simulink model "Car_22_Jan_test_2012b"  (R2012b)
settings: Solver=ode5  StartTime=0.0  StopTime=inf  FixedStep=sample_time  RelTol=1e-3
InitFcn:
  | sample_time=0.005;%0.004;%0.0025;%0.02;
  | sample_time_Vicon = 0.005;
  | DeltaT = 0.02;
  | g = 9.81;
  | H0 = g%0.3165;
  | Kl = 1;
  | 
  | Q6_mass = 0.84;
  | 
  | Q6_Omega_r = 1.5; %for horizon ref
  | Q6_Zeta_r = 0.5; %for horizon ref
  | Q6_Omega_r_h = 2;%for vertical ref
  | Q6_Zeta_r_h = 2; %for vertical ref
  | 
  | 
  | Q6_Omega = 1.5; %for horizon control
  | Q6_Zeta = 0.5; %for horizon control
  | Q6_Omega_h= 2; %for vertical control
  | Q6_Zeta_h = 0.7; %for vertical control
  | 
  | 
  | Q6_acc_max = 5;%horizontal max acc
  | Q6_acc_max_h = 3;%horizontal max acc
  | 
  | omega_circle = 72*pi/180;
  | omega_h = 0.1;%Ascending speed
  | PI = pi;
  | Circle_R = 2.5;
  | MAX_Height = -2;
undefined symbols (not defined in the file): DiscIntNeverNeededParam
libraries: X330_Control x5, dspswit3 x5, simulink x4
(part 2 of 2)

== matlab function Car_22_Jan_test_2012b/UAV 1/Trajectory Logic/trackbounded ==
  data: posx input; posy input; cpx input; cpy input; region output; cvx input; cvy input; newx output; newy output; newregion output; estsecond input; chkfinalx output; chkfinaly output; chknum output; directionflag output; frontbackflag output
function [region,newx,newy,newregion,chkfinalx,chkfinaly,chknum,directionflag,frontbackflag]  = fcn(posx,posy,cpx,cpy,cvx,cvy,estsecond)
%#codegen
%cp = [cpy,cpx,0];
%cpest = [estrawy, estrawx,0];
%%database of check points
chk0x = -0.4383;
chk0y = -0.9285;
chk1x = 1.047;
chk1y = -0.9693;
chk2x = 1.396;
chk2y = 0.4535;
chk3x = 1.382;
chk3y = 1.505;
chk4x = 1.042;
chk4y = 1.925;
chk5x = 0.3708;
chk5y = 1.821;
%%chk5x = ;
%%chk....
chk0 = [chk0y,chk0x,0];
chk1 = [chk1y,chk1x,0];
chk2 = [chk2y,chk2x,0];
chk3 = [chk3y,chk3x,0];
chk4 = [chk4y,chk4x,0];
chk5 = [chk5y,chk5x,0];
distance01 = sqrt((chk0y-chk1y)^2+(chk0x-chk1x)^2);
distance12 = sqrt((chk2y-chk1y)^2+(chk2x-chk1x)^2);
distance23 = sqrt((chk2y-chk3y)^2+(chk2x-chk3x)^2);
distance34 = sqrt((chk3y-chk4y)^2+(chk3x-chk4x)^2);
distance45 = sqrt((chk4y-chk5y)^2+(chk4x-chk5x)^2);
%%%%%%%%%%%%%%%%%%%%%%%%%%%%%%%%%%%%%%%%%%%%%%%%%%%%%%%%%%%%%%%%%%%%%%%%%%%%%%%%%%%%%%region selector
if(cpx>-1 && cpx<=0 && cpy>-1 && cpy<=0)
    region = 0;
elseif(cpx>0 && cpx<=1 && cpy>-1 && cpy<=0 )
    region = 1;
elseif(cpx>1 && cpx<=2 && cpy>-1 && cpy<=0 )
    region = 2;
elseif(cpx>1 && cpx<=2 && cpy>0 &&cpy<=1)
    region = 3;
elseif(cpx>1 && cpx<=2 && cpy>1 && cpy<=2)
    region = 4;
elseif(cpx>1 && cpx<=2 &&cpy>2 && cpy<=3)
    region = 5;
elseif(cpx>0 && cpx<=1 && cpy>2 && cpy<=3)
    region = 6;
elseif(cpx>0 && cpx<=1 && cpy>1 && cpy<=2)
    region = 7;
elseif(cpx>0 && cpx<=1 && cpy>-2 && cpy<=-1)
    region = 8;
elseif(cpx>1 && cpx<=2 && cpy>-2 && cpy<=-1)
    region = 9;
else
    region = -1;
end
%%%%%%%%%%%%%%%%%%%%%%%%%%%%%%%%%%%%%%%%%%%%%%%%%%%%%%%%%%%%%%%%%%%%%%%%%%%%%%%%%%%%%%%%%%%%%%%%%%
if(region == 0 || region==1)
    %%%%%%%%%%%%%%%%calculate point to line distance%%%%%%%%%%%
    %a = chk1 - chk0;
   % b = cp - chk0;
    %d = norm(cross(a,b)) / norm(a);
    angle = atan2((chk1x-chk0x),(chk1y-chk0y));
    samplex = chk0x;
    sampley = chk0y;
    zero = 1;

elseif(region == 2)
    %a = chk2 - chk1;
   % b = cp - chk1;
   % d = norm(cross(a,b)) / norm(a);
    angle = atan2((chk2x-chk1x),(chk2y-chk1y));
    zero = 1;
    samplex = chk1x;
    sampley = chk1y;
elseif(region == 3)
    %a = chk3 - chk2;
    %b = cp - chk2;
   % d = norm(cross(a,b)) / norm(a);
    angle = atan2((chk3x-chk2x),(chk3y-chk2y));
    zero = 1;
    samplex = chk2x;
    sampley = chk2y;
elseif(region == 4 || region==5)
   % a = chk4 - chk3;
   % b = cp - chk3;
    %d = norm(cross(a,b)) / norm(a);
    angle = atan2((chk4x-chk3x),(chk4y-chk3y));
    zero = 1;
      samplex = chk3x;
    sampley = chk3y;
elseif(region == 6 || region==7)
    %a = chk5 - chk4;
    %b = cp - chk4;
    %d = norm(cross(a,b)) / norm(a);
    angle = atan2((chk5x-chk4x),(chk5y-chk4y));
    zero = 1;
      samplex = chk4x;
    sampley = chk4y;
else
    %a = -1;
   % b = -1;
    %d = -1;
    angle = -1;%%% i know this is not correct i will add one more zero coefficient to cancel this case
    zero = 0;
    samplex = 0;
    sampley = 0;
end


%%%%%%%%%%%%%%%%%%%%%%%%%%%%%%%%%%%%%%%%%%%%%%%%%%%%%%%%%%%%%%%%%%%%%%%%%%%%%%%%%%%%%%%%%%%%%%%%%%
% %%calculate project point on the check point line
if(zero == 0)%%if out of boundary none of the region match
        newy = 100;
        newx = 100;
else   %%match the region

        if(angle == 0 ||angle == 180)
            newx  = samplex;
            newy = cpy;
        elseif(angle == 90 || angle == 270)
            newx = cpx;
            newy = sampley;
        else
         kk = -1/(tan(angle));
         m = cpx - kk*cpy ;
         k = tan(angle);
         newy = (samplex - k*sampley - m)/(kk - k);
         newx = kk*newy + m;
         end

end

if(newx>-1 && newx<=0 && newy >-1 && newy <=0)
    newregion = 0;
elseif(newx>0 && newx<=1 && newy>-1 && newy<=0 )
    newregion = 1;
elseif(newx>1 && newx<=2 && newy>-1 && newy<=0 )
    newregion = 2;
elseif(newx>1 && newx<=2 && newy>0 &&newy<=1)
    newregion = 3;
elseif(newx>1 && newx<=2 &&newy>1 && newy<=2)
    newregion = 4;
elseif(newx>1 && newx<=2 &&newy>2 && newy<=3)
    newregion = 5;
elseif(newx>0 && newx<=1 && newy>2 && newy<=3)
    newregion = 6;
elseif(newx>0 && newx<=1 && newy>1 && newy<=2)
    newregion = 7;
elseif(newx>0 && newx<=1 && newy>-2 && newy<=-1)
    newregion = 8;
elseif(newx>1 && newx<=2 && newy>-2 && newy<=-1)
    newregion = 9;
else
    newregion = -1;
end
velangle = atan2(cvx,cvy);
diffvelangletoangle = velangle - angle;
velproject = (cvx^2 + cvy^2)*cos(diffvelangletoangle);
estdistance = estsecond * velproject;
vxyM = sqrt(cvx^2 + cvy^2);
cosdiffvelangletoangle = cos(diffvelangletoangle);
if(vxyM == 0)
    directionflag = 0;
else
if(cosdiffvelangletoangle>=0)
    directionflag = 1;
else
    directionflag = -1;
end
uavcarvectorangle = atan2((posx-cpx),(posy-cpy));
diffuavcartoangle = uavcarvectorangle - angle;
cosdiffuavcartoangle = cos(diffuavcartoangle);
if(cosdiffuavcartoangle>=0)
    frontbackflag = 1;
else
    frontbackflag = 0;
end
end
if(newregion == 0||newregion==1)
    newdistancetonext = sqrt((newy-chk1y)^2+(newx-chk1x)^2);
    if(estdistance < (newdistancetonext))
        chkfinalx = chk1x;
        chkfinaly = chk1y;
        chknum = 1;
    elseif(estdistance>=(newdistancetonext) && estdistance <((newdistancetonext) + distance12))
        chkfinalx = chk2x;
        chkfinaly = chk2y;
        chknum = 2;
    elseif(estdistance>=((newdistancetonext)+distance12)&&estdistance<((newdistancetonext)+distance12+distance23))
        chkfinalx = chk3x;
        chkfinaly = chk3y;
        chknum = 3;
    elseif(estdistance>=((newdistancetonext)+distance12+distance23)&&estdistance<((newdistancetonext)+distance12+distance23+distance34))
        chkfinalx = chk4x;
        chkfinaly = chk4y;
        chknum = 4;
    elseif(estdistance>=((newdistancetonext)+distance12+distance23+distance34)&&estdistance<((newdistancetonext)+distance12+distance23+distance34+distance45))
        chkfinalx = chk5x;
        chkfinaly = chk5y;
        chknum = 5;
    
    else
        chkfinalx = chk5x;
        chkfinaly = chk5y;
        chknum = 5;
    end
elseif(newregion == 2)
    newdistancetonext = sqrt((newy-chk2y)^2+(newx-chk2x)^2);
    if(estdistance < (newdistancetonext))
        chkfinalx = chk2x;
        chkfinaly = chk2y;
        chknum = 2;
    elseif(estdistance >=(newdistancetonext)&&estdistance < ((newdistancetonext)+distance23))
        chkfinalx = chk3x;
        chkfinaly = chk3y;
        chknum = 3;
    elseif(estdistance >=((newdistancetonext)+distance23)&&estdistance < ((newdistancetonext)+distance23+distance34))
        chkfinalx = chk4x;
        chkfinaly = chk4y;
        chknum = 4;
    elseif(estdistance >=((newdistancetonext)+distance23+distance34)&&estdistance < ((newdistancetonext)+distance23+distance34+distance45))
        chkfinalx = chk5x;
        chkfinaly = chk5y;
        chknum = 5;
    else
        chkfinalx = chk5x;
        chkfinaly = chk5y;
        chknum = 5;
    end
elseif(newregion == 3)
    newdistancetonext = sqrt((newy-chk3y)^2+(newx-chk3x)^2);
    if(estdistance < (newdistancetonext))
        chkfinalx = chk3x;
        chkfinaly = chk3y;
        chknum = 3;
    elseif((estdistance >= (newdistancetonext))&&estdistance<((newdistancetonext)+distance34))
        chkfinalx = chk4x;
        chkfinaly = chk4y;
        chknum = 4;
    elseif((estdistance >= (newdistancetonext)+distance34)&&estdistance<((newdistancetonext)+distance34+distance45))
        chkfinalx = chk5x;
        chkfinaly = chk5y;
        chknum = 5;
    else
        chkfinalx = chk5x;
        chkfinaly = chk5y;
        chknum = 5;
    end
elseif(newregion == 4 || newregion == 5)
    newdistancetonext = sqrt((newy-chk4y)^2+(newx-chk4x)^2);
    if(estdistance < (newdistancetonext))
        chkfinalx = chk4x;
        chkfinaly = chk4y;
        chknum = 4;
    elseif((estdistance >= (newdistancetonext))&&estdistance<((newdistancetonext)+distance45))
        chkfinalx = chk5x;
        chkfinaly = chk5y;
        chknum = 5;
    else
        chkfinalx = chk5x;
        chkfinaly = chk5y;
        chknum = 5;
    end
elseif(newregion == 6 || newregion == 7)
    newdistancetonext = sqrt((newy-chk5y)^2+(newx-chk5x)^2);
    if(estdistance < (newdistancetonext))
        chkfinalx = chk5x;
        chkfinaly = chk5y;
        chknum = 5;
    else
        chkfinalx = chk5x;
        chkfinaly = chk5y;
        chknum = 5;
    end
else
    newdistancetonext = -1;
    chkfinalx = 0;
    chkfinaly = 0;
    chknum = -1;
    
end




end
